simulink model "ballTracking"  (R2019b)
settings: Solver=VariableStepAuto  StartTime=0.0  StopTime=2.8  FixedStep=0.0066666666666666666  RelTol=1e-3
PreLoadFcn:
  | addpath(genpath('Video Files'));
undefined symbols (not defined in the file or in its folder): gray
libraries: visiontextngfix x2, visionstatistics x1, dspvision x1
settings Model: Creator=valakshe  LastModifiedBy=valakshe

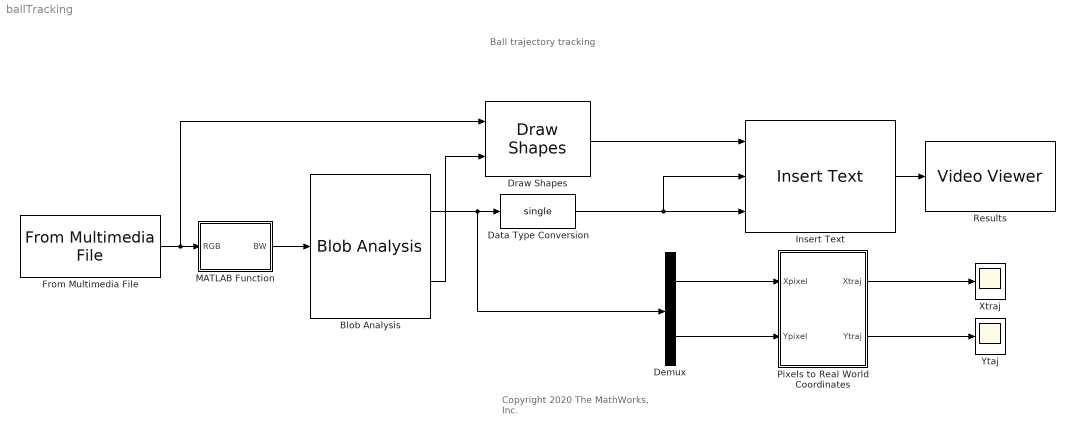
== system ballTracking ==
  note: Copyright 2020 The MathWorks, Inc.
  note: Ball trajectory tracking
  Blob Analysis : visionstatistics/Blob Analysis  Tag=vipblks_row_conv  area=off  centroid=on  bBox=on  majorAxis=off  minorAxis=off  angle=off  eccentricity=off  equivDiameterSq=off  extent=off  perimeter=off  outDT=double  conn=4  isLabel=off  maxBlobs=1  warnIfNumBlobsExceeded=off  isCount=off  useMinArea=on  minArea=2000  useMaxArea=on  maxArea=50000  excludeBorderBlob=off  isOutVarDim=off  isFill=on  fillValues=-1  roundingMode=Floor  overflowMode=off  prodOutputMode=Binary point scaling  prodOutputWordLength=32  prodOutputFracLength=16  prodOutputSlope=2^-16  accumMode=Binary point scaling  accumWordLength=32  accumFracLength=0  accumSlope=2^0  outputMode=Binary point scaling  outputWordLength=32  outputFracLength=16  outputSlope=2^-16  memorySlope=2^-16  firstCoeffMode=Binary point scaling  firstCoeffWordLength=16  firstCoeffFracLength=14  firstCoeffSlope=2^-14  secondCoeffMode=Binary point scaling  secondCoeffWordLength=32  secondCoeffFracLength=16  secondCoeffSlope=2^-16
      settings: SourceProductName=Computer Vision System Toolbox
  Data Type Conversion : DataTypeConversion  OutDataTypeStr=single
  Demux : Demux  Outputs=2
  Draw Shapes : visiontextngfix/Draw Shapes  shape=Rectangles  fill=off  lineWidth=5  fillClrSource=Specify via dialog  display=User-specified value  intensity=200  color=[256 0 0]  opacity=0.6  viewport=Entire image  antialiasing=off  inType=Obsolete  imagePorts=One multidimensional signal  roundingMode=Floor  overflowMode=off  memoryMode=Specify word length  memoryWordLength=16  prodOutputMode=Binary point scaling  prodOutputWordLength=32  prodOutputFracLength=14  prodOutputSlope=2^-14  accumSlope=2^-14  memoryFracLength=15
      settings: SourceProductName=Computer Vision Toolbox
  From Multimedia File : dspvision/From Multimedia File  inputFilename=ballDropping.mp4  readRange=[1 Inf]  loop=on  numPlays=inf  outputStreams=Video only  videoDataType=double  audioDataType=int16  inheritSampleTime=on  userDefinedSampleTime=1/30  noAudioOutput=off  isIntensityVideo=off  fourcc=RGB  colorVideoFormat=One multidimensional signal  outputEOF=off  dataOrg=Column-major  audioFrameSize=1024  computeAudioFrameSize=off  outSamplingMode=Sample based
      settings: SourceProductName=DSP System Toolbox  SourceProductBaseCode=DS
  Insert Text : visiontextngfix/Insert Text  inputType=Obsolete  theText='%0.5f , %0.5f'  getTextLocFrom=Input port  textLoc=[720/2 1280/2]  getTextColorFrom=Specify via dialog  textColor=[0 0 255]  getTextIntensityFrom=Specify via dialog  textIntensity=0  getTextOpacityFrom=Specify via dialog  textOpacity=1.0  dummyVar2=0  dummyVar3=0  dummyVar4=0  imagePorts=One multidimensional signal  isInputTransposed=off  fontFace=LucidaSansRegular  dummyVar1=0  blockFontSize=26  antiAliased=off
      settings: SourceProductName=Computer Vision Toolbox  SourceProductBaseCode=VP
  MATLAB Function : MATLAB Function  TreatAsAtomicUnit=on
  Pixels to Real World Coordinates : Subsystem
  Results : VideoViewer  colormapValue=gray(256)  FigPos=[58 645 479 446]  trueSizedOnce=on
  Xtraj : Scope
  Ytaj : Scope
  wires:
  MATLAB Function/1(BW) -> Blob Analysis/1
  Blob Analysis/2 -> Draw Shapes/2
  From Multimedia File/1 -> Draw Shapes/1, MATLAB Function/1(RGB)
  Draw Shapes/1 -> Insert Text/1
  Insert Text/1 -> Results/1
  Blob Analysis/1 -> Demux/1, Data Type Conversion/1
  Data Type Conversion/1 -> Insert Text/2, Insert Text/3
  Demux/1 -> Pixels to Real World Coordinates/1(Xpixel)
  Demux/2 -> Pixels to Real World Coordinates/2(Ypixel)
  Pixels to Real World Coordinates/1(Xtraj) -> Xtraj/1
  Pixels to Real World Coordinates/2(Ytraj) -> Ytaj/1

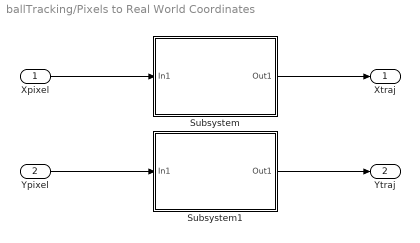
== system ballTracking/Pixels to Real World Coordinates ==
  Xpixel : Inport
  Ypixel : Inport  Port=2
  Subsystem : Subsystem
  Subsystem1 : Subsystem
  Xtraj : Outport
  Ytraj : Outport  Port=2
  wires:
  Xpixel/1 -> Subsystem/1(In1)
  Ypixel/1 -> Subsystem1/1(In1)
  Subsystem1/1(Out1) -> Ytraj/1
  Subsystem/1(Out1) -> Xtraj/1

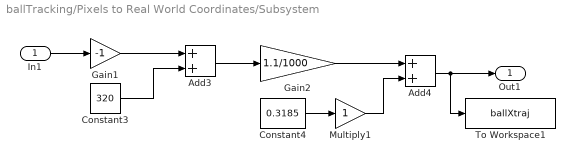
== system ballTracking/Pixels to Real World Coordinates/Subsystem ==
  In1 : Inport
  Add3 : Sum
  Add4 : Sum
  Constant3 : Constant  Value=320
  Constant4 : Constant  Value=0.3185
  Gain1 : Gain  Gain=-1
  Gain2 : Gain  Gain=1.1/1000
  Multiply1 : Gain
  To Workspace1 : ToWorkspace  VariableName=ballXtraj  SampleTime=-1
      settings: Save2DSignal=2-D array (concatenate along first dimension)
  Out1 : Outport
  wires:
  In1/1 -> Gain1/1
  Constant3/1 -> Add3/2
  Gain1/1 -> Add3/1
  Add3/1 -> Gain2/1
  Multiply1/1 -> Add4/2
  Gain2/1 -> Add4/1
  Constant4/1 -> Multiply1/1
  Add4/1 -> Out1/1, To Workspace1/1

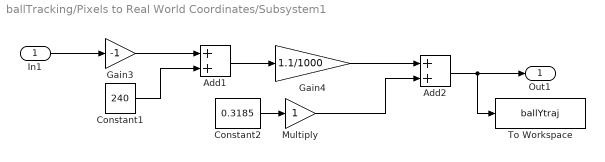
== system ballTracking/Pixels to Real World Coordinates/Subsystem1 ==
  In1 : Inport
  Add1 : Sum
  Add2 : Sum
  Constant1 : Constant  Value=240
  Constant2 : Constant  Value=0.3185
  Gain3 : Gain  Gain=-1
  Gain4 : Gain  Gain=1.1/1000
  Multiply : Gain
  To Workspace : ToWorkspace  VariableName=ballYtraj  SampleTime=-1
      settings: Save2DSignal=2-D array (concatenate along first dimension)
  Out1 : Outport
  wires:
  In1/1 -> Gain3/1
  Multiply/1 -> Add2/2
  Constant1/1 -> Add1/2
  Gain3/1 -> Add1/1
  Add1/1 -> Gain4/1
  Gain4/1 -> Add2/1
  Constant2/1 -> Multiply/1
  Add2/1 -> To Workspace/1, Out1/1

== matlab function ballTracking/MATLAB Function ==
  data: RGB input; BW output
function BW  = createMask(RGB)


% Convert RGB image to chosen color space
I = rgb2lab(RGB);

% Define thresholds for channel 1 based on histogram settings
channel1Min = 11.905;
channel1Max = 93.427;

% Define thresholds for channel 2 based on histogram settings
channel2Min = -19.872;
channel2Max = -4.610;

% Define thresholds for channel 3 based on histogram settings
channel3Min = 14.220;
channel3Max = 61.426;

% Create mask based on chosen histogram thresholds
sliderBW = (I(:,:,1) >= channel1Min ) & (I(:,:,1) <= channel1Max) & ...
    (I(:,:,2) >= channel2Min ) & (I(:,:,2) <= channel2Max) & ...
    (I(:,:,3) >= channel3Min ) & (I(:,:,3) <= channel3Max);
BW = sliderBW;
